simulink model "TelemedicineSync"  (R2026a)
settings: Solver=FixedStepDiscrete  StopTime=100  FixedStep=0.01
undefined symbols (not defined in the file or in its folder): DiscIntNeverNeededParam
libraries: simulink x1

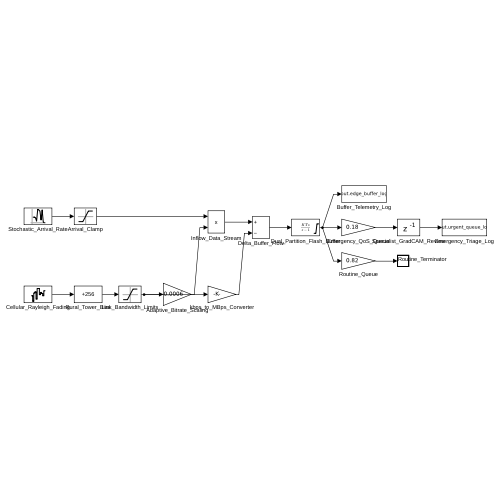
[thumbnail: Simulink's stored preview of the top-level diagram]
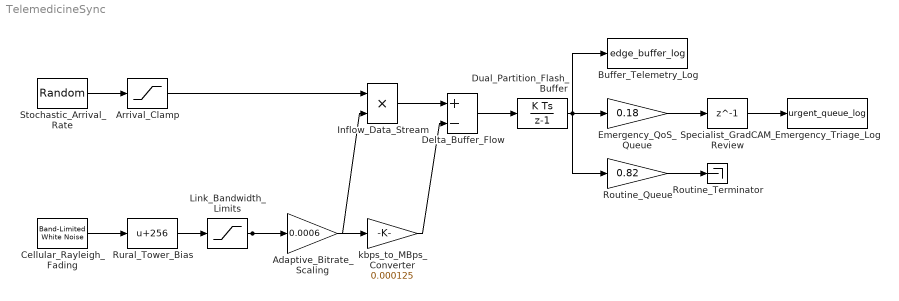
== system TelemedicineSync ==
  Adaptive_Bitrate_Scaling : Gain  Gain=0.0006
  Arrival_Clamp : Saturate  UpperLimit=8.0  LowerLimit=0.5
  Buffer_Telemetry_Log : ToWorkspace  VariableName=edge_buffer_log  SampleTime=-1
  Cellular_Rayleigh_Fading : simulink/Sources/Band-Limited White Noise  Cov=200  Ts=0.1  seed=[23341]
  Delta_Buffer_Flow : Sum  Inputs=+-
  Dual_Partition_Flash_Buffer : DiscreteIntegrator  SampleTime=0.01  LimitOutput=on  UpperSaturationLimit=256  LowerSaturationLimit=0  ICPrevOutput=DiscIntNeverNeededParam  ICPrevScaledInput=DiscIntNeverNeededParam
  Emergency_QoS_Queue : Gain  Gain=0.18
  Emergency_Triage_Log : ToWorkspace  VariableName=urgent_queue_log  SampleTime=-1
  Inflow_Data_Stream : Product  Inputs=**
  Link_Bandwidth_Limits : Saturate  UpperLimit=1500  LowerLimit=10
  Routine_Queue : Gain  Gain=0.82
  Routine_Terminator : Terminator
  Rural_Tower_Bias : Bias  Bias=256  SaturateOnIntegerOverflow=off
  Specialist_GradCAM_Review : Delay  DelayLength=1
  Stochastic_Arrival_Rate : RandomNumber  Mean=3.5  Variance=1.2  SampleTime=0.1
  kbps_to_MBps_Converter : Gain  Gain=0.000125
  wires:
  Stochastic_Arrival_Rate/1 -> Arrival_Clamp/1
  Arrival_Clamp/1 -> Inflow_Data_Stream/1
  Cellular_Rayleigh_Fading/1 -> Rural_Tower_Bias/1
  Rural_Tower_Bias/1 -> Link_Bandwidth_Limits/1
  Link_Bandwidth_Limits/1 -> Adaptive_Bitrate_Scaling/1, kbps_to_MBps_Converter/1
  Adaptive_Bitrate_Scaling/1 -> Inflow_Data_Stream/2
  Inflow_Data_Stream/1 -> Delta_Buffer_Flow/1
  kbps_to_MBps_Converter/1 -> Delta_Buffer_Flow/2
  Delta_Buffer_Flow/1 -> Dual_Partition_Flash_Buffer/1
  Dual_Partition_Flash_Buffer/1 -> Buffer_Telemetry_Log/1, Emergency_QoS_Queue/1, Routine_Queue/1
  Routine_Queue/1 -> Routine_Terminator/1
  Emergency_QoS_Queue/1 -> Specialist_GradCAM_Review/1
  Specialist_GradCAM_Review/1 -> Emergency_Triage_Log/1
